simulink model "Stateflow_actioncondition"  (R2015b)
settings: Solver=VariableStepAuto  StartTime=0.0  StopTime=10.0  RelTol=1e-3
settings Model: Creator=amyyang  LastModifiedBy=amyyang

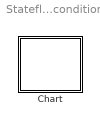
== system Stateflow_actioncondition ==
  Chart : Stateflow chart  TreatAsAtomicUnit=on

== stateflow chart Stateflow_actioncondition/Chart ==
  note: 正确
  note: 错误
  state Correct
  state ?
  state Correct1
  state ?
  state ?
  state ?
  state InCorrect2
  state ?
  state InCorrect3
  state ?
  state ?
  state ?
  state A
  state B
  (default) -> (junction 19) [order 1]
  (default) -> (junction 35) [order 2]
  (junction 19) -> (junction 21) [order 1] : [C1]
  (junction 35) -> (junction 33) [order 2] : [C1]
  (junction 19) -> (junction 20) [order 2] : {
      | out = 0;
      | }
  (junction 35) -> (junction 39) [order 1] : {
      | out = 0;
      | }
  (junction 21) -> (junction 22) : {
      |  out = 1;
      | }
  (junction 33) -> (junction 36) : {
      |  out = 1;
      | }
  (junction 22) -> (junction 20)
  (junction 36) -> (junction 39)
  (junction 20) -> (junction 23)
  (junction 39) -> (junction 37)
  Correct -> ? [order 2]
  Correct -> ? [order 1] : [ u1==1]
  Correct1 -> (junction 52)
  (junction 52) -> ? [order 2]
  (junction 52) -> ? [order 1] : [ u1==1]
  InCorrect2 -> ? [order 1]
  InCorrect2 -> ? [order 2] : [ u1==1]
  InCorrect3 -> (junction 64)
  (junction 64) -> ? [order 1]
  (junction 64) -> ? [order 2] : [ u1==1]
  A -> B : {
      | action;
      | action2;
      | }
